simulink model "EcoSIM3_P2_C2_WIP"  (R2014b)
settings: Solver=ode1  SolverMode=SingleTasking  StartTime=0.0  StopTime=inf  FixedStep=0.01  RelTol=1e-3
PostLoadFcn:
  | %, if any(exist('dsrtsu_mdlpostloadfcn', 'file') == [2, 3, 6]), try dsrtsu_mdlpostloadfcn('Execute', bdroot); catch fprintf('Error in PostLoadFcn (dsrtsu_mdlpostloadfcn) for model "%s":\n %s\n', bdroot, lasterr); end, end,
InitFcn:
  | tic
  | %Startup_EcoSIM
values from neighbouring files (symbols this model uses):
  EngPwr = [0 5	10	15	20	25	30	35	40	45	50	55	60	65	70	75	80	85	90	95	100	105	110	115]    [Series_Maps.m]
  EngSpd = [0 477.4645 954.929 1909.858 2864.787 3819.716 4774.645 5729.574 6684.503]    [Series_Maps.m]
  EngTrq = [0	0	0	0	0	0	0	0	0	0	0	0	0	0	0	0	0	0	0	0	0	0	0	0 ... (first row only)    [Series_Maps.m]
  Power = [0 5 10 15 20 25 30]    [Series_Maps.m]
  Torque = [-50,-40,-30,-25,-20,-15,-10,-8,-6,-4,-2,0]    [Series_Maps.m]
undefined symbols (not defined in the file or in its folder): canChannel, Controls, DriveCycles, Driver, EM_EFF_MAP, EM_PwrLoss_MAP, Glbl, Overwritten_Mode, Plants, sigbuilder_block, Trialmap, Veh_Dynamics
libraries: simulink x141, canmsglib x113, fl_lib x104, canlib x89, nesl_utility x56, sdl_lib x29, dspsigops x6, dspswit3 x5, dspstat3 x2, commnoisgen2 x1, dspfdesign x1
(part 21 of 21)

== stateflow chart EcoSIM3_P2_C2_WIP/Supervisory Controller/Mode Operation/Limited EV/Temperature Limiting Disbuf/Chart1 ==
  state Init
    en, du: EM_trq = trq_request;
  state ModifiedSplit
    en, du: EM_trq = trq_split_in*trq_request;
    ICE_trq = (1-trq_split_in)*trq_request;
  (default) -> Init
  ModifiedSplit -> Init : [(1-trq_split_in)*trq_request < eng_trq_thres_off]
  Init -> ModifiedSplit : [(1-trq_split_in)*trq_request >= eng_trq_thres_on]
  data: EM_trq output; trq_split_in input; eng_trq_thres_on input; eng_trq_thres_off input; trq_request input; ICE_trq output

== stateflow chart EcoSIM3_P2_C2_WIP/Supervisory Controller/Mode Operation/Limited EV/ICE_torque/Trans Clutch Messages/GentleClutchRelease ==
  state Entry
    entry: Shift_Request=0;
  state EngagementTransition
    entry: Shift_Request=0;
    exit: Shift_Request=0;
    state LowSpeed
      entry: Shift_Request=0;
    state Transition
      entry: Shift_Request=1.5*(BAS_Speed-Lower_Clutch_Speed);
      during: Shift_Request=1.5*(BAS_Speed-Lower_Clutch_Speed);
    state FullyEngaged
      entry: Shift_Request=100;
    (default) -> LowSpeed
    Transition -> LowSpeed [order 1] : [BAS_Speed<=Lower_Clutch_Speed]
    FullyEngaged -> LowSpeed [order 1] : [BAS_Speed<=Lower_Clutch_Speed]
    LowSpeed -> Transition : [BAS_Speed>Lower_Clutch_Speed]
    Transition -> FullyEngaged [order 2] : [BAS_Speed>=Upper_Clutch_Speed]
    FullyEngaged -> Transition [order 2] : [BAS_Speed<Upper_Clutch_Speed]
  (default) -> Entry
  EngagementTransition -> Entry : [Clutch_Request==0]
  Entry -> EngagementTransition : [Clutch_Request==1]
  data: BAS_Speed input; Clutch_Request input; Lower_Clutch_Speed input; Upper_Clutch_Speed input; Shift_Request output

== stateflow chart EcoSIM3_P2_C2_WIP/Supervisory Controller/Mode Operation/Series1/Engine Torque Request1 ==
  state Entry
    entry: Torque_Request=0;
  state TorqueRequest
    state FullTorque
      entry: Torque_Request= 80-2.75*(BAS_Speed-Desired_BAS_Speed);
      during: Torque_Request= 80-2.75*(BAS_Speed-Desired_BAS_Speed);
    state FullTorque1
      entry: Torque_Request= 80;
    FullTorque1 -> FullTorque : [BAS_Speed>Desired_BAS_Speed]
    FullTorque -> FullTorque1 : [BAS_Speed<Desired_BAS_Speed]
    (default) -> FullTorque1
  (default) -> Entry
  TorqueRequest -> Entry : [BAS_Speed>Desired_BAS_Speed+20]
  Entry -> TorqueRequest : [BAS_Speed<530]
  data: BAS_Speed input; Torque_Request output; Desired_BAS_Speed input

== stateflow chart EcoSIM3_P2_C2_WIP/Supervisory Controller/Mode Selection /Start-Stop control/Engine_Start_Stop ==
  state Engine_Start
    en, du: Mode = 4;
    Time_in_wait = 0;
  state Engine_Only
    en, du: Mode = 3;
    Time_in_wait = 0;
  state Engine_Wait_State
    en, du: Mode = 3;
    Time_in_wait = 1;
  state Engine_Stop
    en, du: Mode = 2;
    Time_in_wait = 0;
  (default) -> (junction 38)
  Engine_Stop -> Engine_Start : [Alpha_Percent>2]
  (junction 38) -> Engine_Start [order 2]
  (junction 38) -> Engine_Only [order 1] : [eng_running==1]
  Engine_Start -> Engine_Only : [eng_running==1]
  Engine_Only -> Engine_Wait_State : [Alpha_Percent==0 &&...
      | Vehicle_Speed<=1]
  Engine_Wait_State -> Engine_Only [order 1] : [Alpha_Percent>0&&...
      | Time_to_Stop<Time_in_wait_limit]
  Engine_Wait_State -> Engine_Stop [order 2] : [Time_to_Stop>Time_in_wait_limit]
  data: Vehicle_Speed input; Brake_Pedal_Position input; Alpha_Percent input; eng_running input; Mode output; Time_in_wait output; Time_in_wait_limit input; Time_to_Stop input

== stateflow chart EcoSIM3_P2_C2_WIP/Supervisory Controller/Mode Operation/Engine Only /Trans Clutch Messages/AggressiveClutchRelease ==
  state Entry
    entry: Shift_Request=0;
  state EngagementTransition
    entry: Shift_Request=0;
    exit: Shift_Request=0;
    state LowSpeed
      entry: Shift_Request=0;
    state Transition
      entry: Shift_Request=0.5*(BAS_Speed-Lower_Clutch_Speed);
      during: Shift_Request=0.5*(BAS_Speed-Lower_Clutch_Speed);
    state FullyEngaged
      entry: Shift_Request=100;
    (default) -> LowSpeed
    Transition -> LowSpeed [order 1] : [BAS_Speed<=Lower_Clutch_Speed]
    FullyEngaged -> LowSpeed [order 1] : [BAS_Speed<=Lower_Clutch_Speed]
    LowSpeed -> Transition : [BAS_Speed>185+5]
    Transition -> FullyEngaged [order 2] : [BAS_Speed>=375+5]
    FullyEngaged -> Transition [order 2] : [BAS_Speed<Upper_Clutch_Speed]
  (default) -> Entry
  EngagementTransition -> Entry : [Clutch_Request==0]
  Entry -> EngagementTransition : [Clutch_Request==1]
  data: BAS_Speed input; Clutch_Request input; Lower_Clutch_Speed input; Upper_Clutch_Speed input; Shift_Request output

== stateflow chart EcoSIM3_P2_C2_WIP/Powertrain/Accessories Power Module/Subsystem/Algorithm/CAN fault ==
  state Normal
    entry:
    CANdown=0;
    count=0;
    state=1;
  state Abnormal
    entry:
    count=1;
    state=2;
    during:
    count=count+1;
  state Fault
    entry:
    CANdown=1;
    state=0;
  (default) -> Normal
  Normal -> Abnormal : [LowVoltEnblRq ~=0 && LowVoltEnblRq ~=1 && PowerUp>0]
  Fault -> Normal : [PowerUp==0]
  Abnormal -> Normal [order 2] : [LowVoltEnblRq ==0 || LowVoltEnblRq ==1]
  Abnormal -> Fault [order 1] : [count>=10]
  data: CANdown output; PowerUp input; LowVoltEnblRq input; count local; state output

== stateflow chart EcoSIM3_P2_C2_WIP/Powertrain/Accessories Power Module/Subsystem/Algorithm/DC-DC SoftECU ==
  state Working
    state Enable
      entry:
      AccPwrMdlLowVlt=0;
      AccPwrMdlLwVltSysFld=0;
      State=2;
      during:
    state Operation
      entry:
      AccPwrMdlLowVlt=LwVltStpntCmnd;
      AccPwrMdlLwVltSysFld=0;
      State=3;
      during:
      AccPwrMdlLowVlt=LwVltStpntCmnd;
    (default) -> Enable
    Operation -> Enable : [LowVoltEnblRq==0]
    Enable -> Operation : [LowVoltEnblRq==1]
  state Off
    entry:
    AccPwrMdlLowVlt=0;
    AccPwrMdlLwVltSysFld=0;
    State=1;
  state Fault
    entry:
    AccPwrMdlLowVlt=0;
    AccPwrMdlLwVltSysFld=1;
    State=0;
    during:
  Working -> Fault [order 1] : [Fault==1 || CANdown==1]
  Off -> Working [order 2] : [PowerUp>0  && bcm_mainc_stat==1]
  Working -> Off [order 2] : [PowerUp==0  || bcm_mainc_stat==0]
  (default) -> Off
  Off -> Fault [order 1] : [Fault==1]
  Fault -> Off : [Fault==0 && PowerUp==0]
  data: CANdown input; State output; PowerUp input; LowVoltEnblRq input; bcm_mainc_stat input; LwVltStpntCmnd input; Fault input boolean; bcmVbat input; PowerReq input; AccPwrMdlLowVlt output; AccPwrMdlLwVltSysFld output

== stateflow chart EcoSIM3_P2_C2_WIP/Powertrain/Accessories Power Module/Plant/Chart ==
  state Inactive
    entry:
    APMLwVltOtptCrntUns=0;
    AccPwrMdlHiVltInpCrnt=0;
  state Active
    entry:
    APMLwVltOtptCrntUns=PowerReq/AccPwrMdlLowVlt;
    AccPwrMdlHiVltInpCrnt=PowerReq/bcmVbat/.98;
    during:
    APMLwVltOtptCrntUns=PowerReq/AccPwrMdlLowVlt;
    AccPwrMdlHiVltInpCrnt=PowerReq/bcmVbat/.98;
  (default) -> Inactive
  Inactive -> Active : [AccPwrMdlLowVlt~=0]
  data: APMLwVltOtptCrntUns output; AccPwrMdlHiVltInpCrnt output; AccPwrMdlLowVlt input; PowerReq input; bcmVbat input
